simulink model "PMSM_DTC_improved"  (R2022b)
settings: Solver=ode3  StartTime=0.0  StopTime=0.6  FixedStep=5e-6  MaxStep=1e-3  RelTol=1e-4  EnableMultiTasking=on
InitFcn:
  | clear all;
libraries: spsDCVoltageSourceLib x2, spsGroundLib x2, spsPermanentMagnetSynchronousMachineLib x2, spsThreePhaseVIMeasurementLib x2, spsUniversalBridgeLib x2, simulink x1, spsTriangleGeneratorLib x1, sps_lib x1
settings Model: Creator=Administrator  LastModifiedBy=86135
settings SolverCC: AlgebraicLoopSolver=TrustRegion  SolverResetMethod=Robust
settings DataIOCC: LimitDataPoints=on  SaveFormat=Array  SignalLoggingSaveFormat=ModelDataLogs  ReturnWorkspaceOutputs=off
settings OptimizationCC: ExpressionDepthLimit=2147483647  InitFltsAndDblsToZero=on  LifeSpan=inf
settings DebuggingCC: UnderspecifiedInitializationDetection=Classic  MergeDetectMultiDrivingBlocksExec=none  SolverPrmCheckMsg=warning  FcnCallInpInsideContextMsg=warning  UnconnectedInputMsg=warning  UnconnectedOutputMsg=warning  UnconnectedLineMsg=warning  StateNameClashWarn=warning  SFUnexpectedBacktrackingDiag=warning  SFNoUnconditionalDefaultTransitionDiag=warning  SFExecutionAtInitializationDiag=none  SFMachineParentedDataDiag=warning  ArithmeticOperatorsInVariantConditions=warning
settings HardwareCC: ProdBitPerPointer=32  ProdBitPerSizeT=32  ProdBitPerPtrDiffT=32  ProdLargestAtomicFloat=None  ProdIntDivRoundTo=Undefined  ProdEndianess=Unspecified  ProdWordSize=32  ProdHWDeviceType=32-bit Generic
settings ModelReferenceCC: PropagateSignalLabelsOutOfModel=off
settings SFSimCC: SimUseLocalCustomCode=off  CustomCodeUndefinedFunction=UseInterfaceOnly
settings RTWCC: RTWUseLocalCustomCode=off
settings CodeAppCC: StateflowObjectComments=on
settings GRTTargetCC: TargetLangStandard=C89/C90 (ANSI)  CombineOutputUpdateFcns=off  GRTInterface=on
settings ConfigComp: CovMetricSettings=dw  CovSaveCumulativeToWorkspaceVar=on  CovSaveSingleToWorkspaceVar=on  CovExternalEMLEnable=off  CovSFcnEnable=off
settings SimscapeCC: SimscapeNormalizeSystem=off

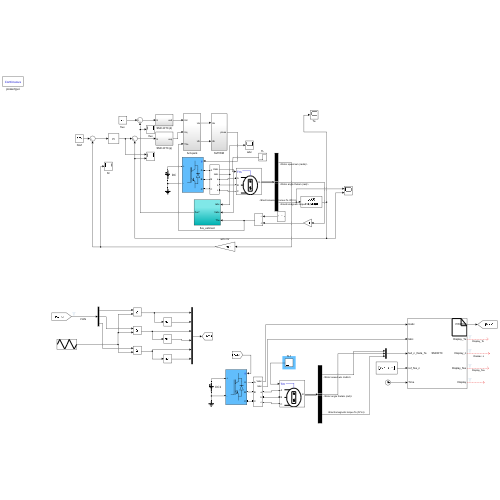
[thumbnail: Simulink's stored preview of the top-level diagram]
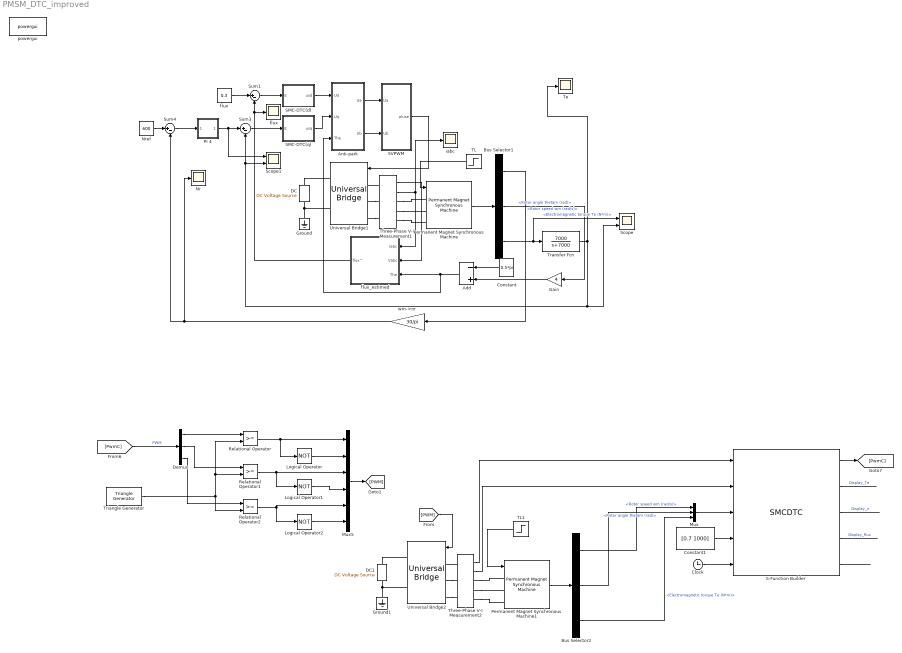
== system PMSM_DTC_improved ==
  Add : Sum  Inputs=-+
  Anti-park : Subsystem
  Bus Selector1 : BusSelector  OutputSignals=Rotor speed wm (rad/s),Rotor angle thetam (rad),Electromagnetic torque Te (N*m)
  Bus Selector2 : BusSelector  OutputSignals=Rotor speed wm (rad/s),Rotor angle thetam (rad),Electromagnetic torque Te (N*m)
  Clock : Clock
  Constant : Constant  Value=0.5*pi
  Constant1 : Constant  Value=[0.7 1000]
  DC : spsDCVoltageSourceLib/DC Voltage Source  Amplitude=311  Measurements=None
  DC1 : spsDCVoltageSourceLib/DC Voltage Source  Amplitude=500  Measurements=None
  Demux : Demux  Outputs=3
  Gain : Gain  Gain=4
  Ground : spsGroundLib/Ground  LConnTagsString=a
  Ground1 : spsGroundLib/Ground  LConnTagsString=a
  Logical Operator : Logic  Operator=NOT  AllPortsSameDT=off  OutDataTypeStr=boolean
  Logical Operator1 : Logic  Operator=NOT  AllPortsSameDT=off  OutDataTypeStr=boolean
  Logical Operator2 : Logic  Operator=NOT  AllPortsSameDT=off  OutDataTypeStr=boolean
  Mux : Mux  Inputs=3
  Mux5 : Mux  Inputs=6
  Nr : Scope
  Nref : Constant  Value=600
  PI 4 : Subsystem
      mask Display: disp('PI')
  Permanent Magnet Synchronous Machine : spsPermanentMagnetSynchronousMachineLib/Permanent Magnet Synchronous Machine  NbPhases=3  FluxDistribution=Sinusoidal  RotorType=Salient-pole  MechanicalLoad=Torque Tm  PresetModel=No  ShowDetailedParameters=on  MeasurementBus=off  Resistance=1.2  Inductance=8.5e-3  dqInductances=[8.5e-3,8.5e-3]  La=0.000835  MachineConstant=Torque Constant (N.m / A_peak)  Flux=0.175  VoltageCst=126.966  TorqueCst=1.05  Flat=120  Mechanical=[0.0008 0 4]  PolePairs=4  InitialConditions=[0,0, 0,0]  InitialConditions5ph=[0 0 0 0 0 0]  RefAngle=90 degrees behind phase A axis (modified Park)  IterativeDiscreteModel=Trapezoidal non iterative  TsBlock=-1  TsPowergui=0
  Permanent Magnet Synchronous Machine1 : spsPermanentMagnetSynchronousMachineLib/Permanent Magnet Synchronous Machine  NbPhases=3  FluxDistribution=Sinusoidal  RotorType=Salient-pole  MechanicalLoad=Torque Tm  PresetModel=No  ShowDetailedParameters=on  MeasurementBus=off  Resistance=1.2  Inductance=8.5e-3  dqInductances=[8.5e-3,8.5e-3]  La=0.000835  MachineConstant=Torque Constant (N.m / A_peak)  Flux=0.175  VoltageCst=126.966  TorqueCst=1.05  Flat=120  Mechanical=[0.0008 0 4]  PolePairs=4  InitialConditions=[0,0, 0,0]  InitialConditions5ph=[0 0 0 0 0 0]  RefAngle=90 degrees behind phase A axis (modified Park)  IterativeDiscreteModel=Trapezoidal non iterative  TsBlock=-1  TsPowergui=0
  Relational Operator : RelationalOperator  OutDataTypeStr=boolean  RndMeth=Simplest  InputSameDT=off
  Relational Operator1 : RelationalOperator  OutDataTypeStr=boolean  RndMeth=Simplest  InputSameDT=off
  Relational Operator2 : RelationalOperator  OutDataTypeStr=boolean  RndMeth=Simplest  InputSameDT=off
  S-Function Builder : S-Function  FunctionName=SMCDTC  SFunctionModules=SMCDTC_wrapper.c ControlFunction InverterController  SFunctionDeploymentMode=off  EnableBusSupport=off  mask(S-Function Builder){}
      mask help: Simulink:masks:SFunctionBuilder_MD
      mask init:
      | val = [[.9  0.75 0.75 1 1 .9 .9 1]',[1 1 0.75 0.75 .9 .9 1 .9]'];try , sys = get_param(gcb,'SfunBuilderFcnName');if isempty(sys), sys = get_param(gcb,'FunctionName'); end,catch, sys = get_param(gcb,'FunctionName'); end
      settings: CopyFcn=set_param(gcbh,'LinkStatus','none')  OpenFcn=sfunctionwizard(gcbh)
      mask Display:
      | plot(val(:,1),val(:,2))
      | disp(sys)
      | port_label('input',1,'Uabc')
      | port_label('input',2,'Iabc')
      | port_label('input',3,'fed_n_theta_Te')
      | port_label('input',4,'ref_flux_n')
      | port_label('input',5,'Time')
      | port_label('output',1,'PWMRef')
      | port_label('output',2,'Display_Te')
      | port_label('output',3,'Display_n')
      | port_label('output',4,'Display_flux')
      | port_label('output',5,'Display')
  SMC-DTC(d) : Subsystem
  SMC-DTC(q) : Subsystem
  SVPWM : Subsystem
  Scope : Scope  NumInputPorts=2
  Scope1 : Scope  NumInputPorts=2
  Sum1 : Sum  Inputs=|+-
  Sum3 : Sum  Inputs=|+-
  Sum4 : Sum  Inputs=|+-
  TL : Step  Time=0.2  After=1.5  SampleTime=0
  TL1 : Step  Time=0.2  After=1.3  SampleTime=0
  Te : Scope
  Three-Phase V-I Measurement1 : spsThreePhaseVIMeasurementLib/Three-Phase V-I Measurement  VoltageMeasurement=phase-to-ground  SetLabelV=off  LabelV=Vabc  Vpu=off  VpuLL=off  CurrentMeasurement=yes  SetLabelI=off  LabelI=Iabc  Ipu=off  Pbase=100e6  Vbase=500e3  OutputType=Complex  PhasorSimulation=off  PSBequivalent=0
  Three-Phase V-I Measurement2 : spsThreePhaseVIMeasurementLib/Three-Phase V-I Measurement  VoltageMeasurement=phase-to-ground  SetLabelV=off  LabelV=Vabc  Vpu=off  VpuLL=off  CurrentMeasurement=yes  SetLabelI=off  LabelI=Iabc  Ipu=off  Pbase=100e6  Vbase=500e3  OutputType=Complex  PhasorSimulation=off  PSBequivalent=0
  Transfer Fcn : TransferFcn  Numerator=[7000]  Denominator=[1 7000]
  Triangle Generator : spsTriangleGeneratorLib/Triangle Generator  Freq=5e3  Phase=90  Ts=0
  Universal Bridge1 : spsUniversalBridgeLib/Universal Bridge  Arms=3  SnubberResistance=1e5  SnubberCapacitance=inf  Device=IGBT / Diodes  Ron=1e-3  Lon=0  ForwardVoltages="[  0  0  ]"  ForwardVoltage=0  GTOparameters=[ 10e-6 , 20e-6 ]  IGBTparameters=[ 1e-6 , 2e-6 ]  Measurements=None  Measurements_2=None  converterType=Rectifier
  Universal Bridge2 : spsUniversalBridgeLib/Universal Bridge  Arms=3  SnubberResistance=1e5  SnubberCapacitance=inf  Device=IGBT / Diodes  Ron=1e-3  Lon=0  ForwardVoltages="[  0  0  ]"  ForwardVoltage=0  GTOparameters=[ 10e-6 , 20e-6 ]  IGBTparameters=[ 1e-6 , 2e-6 ]  Measurements=None  Measurements_2=None  converterType=Rectifier
  flux : Scope
  "flux " : Constant  Value=0.3
  flux_estimed : Subsystem
  iabc : Scope
  powergui : sps_lib/powergui  SimulationMode=Continuous  SampleTime=50e-6  frequency=60  Iterations=50  frequencyindice=0  Pbase=100e6  ErrMax=1e-4  UnitsV=kV  UnitsW=MW  buscounter=0  FunctionMessages=off  echomessages=off  EnableUseOfTLC=off  CurrentSourceSwitches=off  DisableSnubberDevices=off  DisableRonSwitches=off  DisableVfSwitches=off  DisplayEquations=off  AutomaticDiscreteSolvers=off  SolverType=Tustin/Backward Euler (TBE)  Interpol=off  ExternalGateDelay=off  methode=off  Ts=0  x0status=blocks  SPID=off  SwTol=0  HookPort=off  NonlinearTolerance=1e-4  nMaxIteration=100  ContinueOnMaxIteration=off  RestoreLinks=warning  ResistiveCurrentMeasurement=off  Frange=[0:2:500]  Ylog=off  Xlog=on  ShowGrid=off  save=off  variable=ZData  structure=0  ZoomFFT=on  StartTime=0.0  cycles=1  DisplayStyle=1  fundamental=60  FreqAxis=off  MaxFrequency=1000  frequencyindicesteady=1  RmsSteady=1  display=off
  wm->nr : Gain  Gain=30/pi
  wires:
  Anti-park/1(Ua) -> SVPWM/1(Ua)
  Anti-park/2(Ub) -> SVPWM/2(Ub)
  SMC-DTC(d)/1(usd) -> Anti-park/1(Ud)
  "flux "/1 -> Sum1/1
  Sum1/1 -> SMC-DTC(d)/1(E)
  SMC-DTC(q)/1(usq) -> Anti-park/2(Uq)
  Nref/1 -> Sum4/1
  Sum4/1 -> PI 4/1(In1)
  Sum3/1 -> SMC-DTC(q)/1(E)
  wm->nr/1 -> Sum4/2, Nr/1
  TL/1 -> Permanent Magnet Synchronous Machine/1
  SVPWM/1(pluse) -> Universal Bridge1/1
  flux_estimed/1(flux^) -> Sum1/2, flux/1
  Three-Phase V-I Measurement1/1 -> flux_estimed/2(Vabc)
  Gain/1 -> Add/2
  Constant/1 -> Add/1
  Add/1 -> Anti-park/3(The), flux_estimed/3(The)
  Three-Phase V-I Measurement1/2 -> flux_estimed/1(Iabc), iabc/1
  Bus Selector1/3 -> Scope/1, Transfer Fcn/1  "<Electromagnetic torque Te (N*m)>"
  Bus Selector1/2 -> Gain/1  "<Rotor angle thetam (rad)>"
  Bus Selector1/1 -> wm->nr/1  "<Rotor speed wm (rad/s)>"
  Permanent Magnet Synchronous Machine/1 -> Bus Selector1/1
  Permanent Magnet Synchronous Machine1/1 -> Bus Selector2/1
  Three-Phase V-I Measurement2/2 -> S-Function Builder/2
  Bus Selector2/3 -> Mux/3  "<Electromagnetic torque Te (N*m)>"
  TL1/1 -> Permanent Magnet Synchronous Machine1/1
  Bus Selector2/1 -> Mux/1  "<Rotor speed wm (rad/s)>"
  Three-Phase V-I Measurement2/1 -> S-Function Builder/1
  Demux/1 -> Relational Operator/1
  Mux5/1 -> [PWM]
  Relational Operator1/1 -> Mux5/3, Logical Operator1/1
  Logical Operator/1 -> Mux5/2
  Demux/3 -> Relational Operator2/1
  Triangle Generator/1 -> Relational Operator/2, Relational Operator1/2, Relational Operator2/2
  Demux/2 -> Relational Operator1/1
  Relational Operator2/1 -> Mux5/5, Logical Operator2/1
  Logical Operator1/1 -> Mux5/4
  Logical Operator2/1 -> Mux5/6
  Relational Operator/1 -> Mux5/1, Logical Operator/1
  [PwmC] -> Demux/1  "PWM"
  S-Function Builder/1 -> [PwmC]
  Mux/1 -> S-Function Builder/3
  Bus Selector2/2 -> Mux/2  "<Rotor angle thetam (rad)>"
  Constant1/1 -> S-Function Builder/4
  [PWM] -> Universal Bridge2/1
  Clock/1 -> S-Function Builder/5
  S-Function Builder/2 -> ?  "Display_Te"
  S-Function Builder/3 -> ?  "Display_n"
  S-Function Builder/4 -> ?  "Display_flux"
  S-Function Builder/5 -> ?
  Transfer Fcn/1 -> Te/1, Scope1/2, Sum3/2, Scope/2
  PI 4/1(Out1) -> Scope1/1, Sum3/1
  connections:
  Ground/LConn1 -- Universal Bridge1/RConn2 -- DC/LConn1
  Three-Phase V-I Measurement1/RConn1 -- Permanent Magnet Synchronous Machine/LConn1
  DC/RConn1 -- Universal Bridge1/RConn1
  Universal Bridge1/LConn2 -- Three-Phase V-I Measurement1/LConn2
  Three-Phase V-I Measurement1/LConn1 -- Universal Bridge1/LConn1
  Universal Bridge1/LConn3 -- Three-Phase V-I Measurement1/LConn3
  Three-Phase V-I Measurement1/RConn3 -- Permanent Magnet Synchronous Machine/LConn3
  Three-Phase V-I Measurement1/RConn2 -- Permanent Magnet Synchronous Machine/LConn2
  DC1/LConn1 -- Ground1/LConn1 -- Universal Bridge2/RConn2
  Three-Phase V-I Measurement2/LConn1 -- Universal Bridge2/LConn1
  Three-Phase V-I Measurement2/RConn3 -- Permanent Magnet Synchronous Machine1/LConn3
  Universal Bridge2/LConn2 -- Three-Phase V-I Measurement2/LConn2
  Three-Phase V-I Measurement2/RConn1 -- Permanent Magnet Synchronous Machine1/LConn1
  DC1/RConn1 -- Universal Bridge2/RConn1
  Three-Phase V-I Measurement2/RConn2 -- Permanent Magnet Synchronous Machine1/LConn2
  Universal Bridge2/LConn3 -- Three-Phase V-I Measurement2/LConn3

== system PMSM_DTC_improved/Anti-park ==
  Ud : Inport
  Uq : Inport  Port=2
  The : Inport  Port=3
  Fcn : Fcn  Expr=u(1)*cos(u(3))-u(2)*sin(u(3))
  Fcn1 : Fcn  Expr=u(1)*sin(u(3))+u(2)*cos(u(3))
  Mux1 : Mux  Inputs=3
  Ua : Outport
  Ub : Outport  Port=2
  wires:
  Uq/1 -> Mux1/2
  Ud/1 -> Mux1/1
  Fcn1/1 -> Ub/1
  Fcn/1 -> Ua/1
  Mux1/1 -> Fcn1/1, Fcn/1
  The/1 -> Mux1/3

== system PMSM_DTC_improved/PI 4 ==
  In1 : Inport
  Add : Sum
  Gain : Gain  Gain=0.05
  Gain1 : Gain  Gain=20
  Integrator : Integrator
  Saturation : Saturate  UpperLimit=50  LowerLimit=-50
  Out1 : Outport
  wires:
  Gain1/1 -> Integrator/1
  In1/1 -> Gain/1, Gain1/1
  Gain/1 -> Add/1
  Integrator/1 -> Add/2
  Add/1 -> Saturation/1
  Saturation/1 -> Out1/1

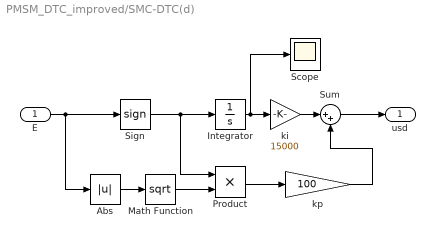
== system PMSM_DTC_improved/SMC-DTC(d) ==
  E : Inport
  Abs : Abs  SaturateOnIntegerOverflow=off
  Integrator : Integrator
  Math Function : Math  Operator=sqrt  SignedPower=on
  Product : Product  RndMeth=Zero
  Scope : Scope
  Sign : Signum
  Sum : Sum  Inputs=|++
  ki : Gain  Gain=15000
  kp : Gain  Gain=100
  usd : Outport
  wires:
  Sum/1 -> usd/1
  E/1 -> Sign/1, Abs/1
  Sign/1 -> Integrator/1, Product/1
  Abs/1 -> Math Function/1
  Math Function/1 -> Product/2
  Product/1 -> kp/1
  kp/1 -> Sum/2
  ki/1 -> Sum/1
  Integrator/1 -> Scope/1, ki/1

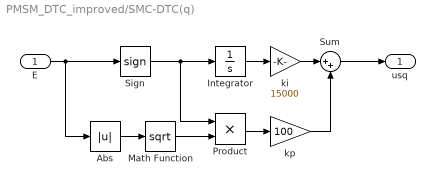
== system PMSM_DTC_improved/SMC-DTC(q) ==
  E : Inport
  Abs : Abs  SaturateOnIntegerOverflow=off
  Integrator : Integrator
  Math Function : Math  Operator=sqrt  SignedPower=on
  Product : Product  RndMeth=Zero
  Sign : Signum
  Sum : Sum  Inputs=|++
  ki : Gain  Gain=15000
  kp : Gain  Gain=100
  usq : Outport
  wires:
  ki/1 -> Sum/1
  kp/1 -> Sum/2
  Product/1 -> kp/1
  Math Function/1 -> Product/2
  Abs/1 -> Math Function/1
  Integrator/1 -> ki/1
  Sign/1 -> Product/1, Integrator/1
  E/1 -> Abs/1, Sign/1
  Sum/1 -> usq/1

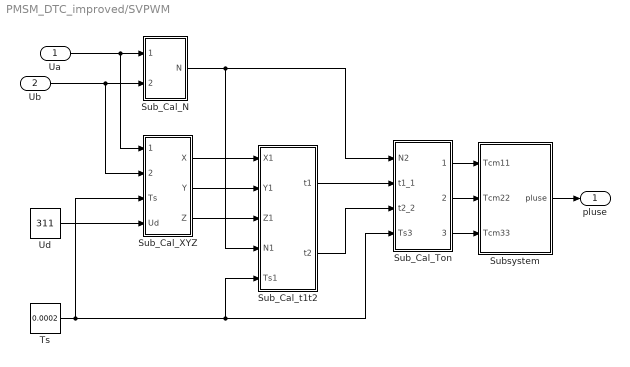
== system PMSM_DTC_improved/SVPWM ==
  Ua : Inport
  Ub : Inport  Port=2
  Sub_Cal_N : Subsystem
  Sub_Cal_Ton : Subsystem
  Sub_Cal_XYZ : Subsystem
  Sub_Cal_t1t2 : Subsystem
  Subsystem : Subsystem
  Ts : Constant  Value=0.0002
  Ud : Constant  Value=311
  pluse : Outport
  wires:
  Ua/1 -> Sub_Cal_N/1(Ualfa), Sub_Cal_XYZ/1(Ualfa1)
  Ub/1 -> Sub_Cal_N/2(Ubeta), Sub_Cal_XYZ/2(Ubeta1)
  Sub_Cal_XYZ/1(X) -> Sub_Cal_t1t2/1(X1)
  Sub_Cal_XYZ/2(Y) -> Sub_Cal_t1t2/2(Y1)
  Sub_Cal_XYZ/3(Z) -> Sub_Cal_t1t2/3(Z1)
  Sub_Cal_t1t2/1(t1) -> Sub_Cal_Ton/2(t1_1)
  Sub_Cal_Ton/1(Tcm1) -> Subsystem/1(Tcm11)
  Sub_Cal_Ton/2(Tcm2) -> Subsystem/2(Tcm22)
  Ts/1 -> Sub_Cal_Ton/4(Ts3), Sub_Cal_t1t2/5(Ts1), Sub_Cal_XYZ/3(Ts)
  Sub_Cal_Ton/3(Tcm3) -> Subsystem/3(Tcm33)
  Subsystem/1(pluse) -> pluse/1
  Sub_Cal_t1t2/2(t2) -> Sub_Cal_Ton/3(t2_2)
  Ud/1 -> Sub_Cal_XYZ/4(Ud)
  Sub_Cal_N/1(N) -> Sub_Cal_Ton/1(N2), Sub_Cal_t1t2/4(N1)

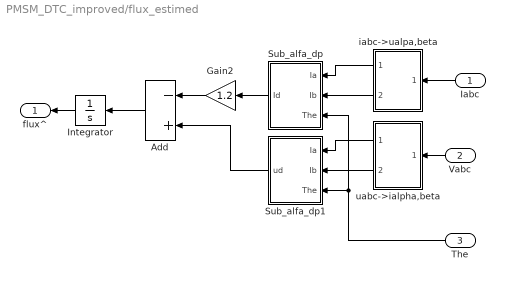
== system PMSM_DTC_improved/flux_estimed ==
  Iabc : Inport
  Vabc : Inport  Port=2
  The : Inport  Port=3
  Add : Sum  Inputs=-+
  Gain2 : Gain  Gain=1.2
  Integrator : Integrator
  Sub_alfa_dp : Subsystem
  Sub_alfa_dp1 : Subsystem
  iabc->ualpa,beta : Subsystem
  uabc->ialpha,beta : Subsystem
  flux^ : Outport
  wires:
  iabc->ualpa,beta/1(ialfa) -> Sub_alfa_dp/1(Ia)
  iabc->ualpa,beta/2(ibeta) -> Sub_alfa_dp/2(Ib)
  uabc->ialpha,beta/1(ualfa) -> Sub_alfa_dp1/1(Ia)
  uabc->ialpha,beta/2(ubeta) -> Sub_alfa_dp1/2(Ib)
  Sub_alfa_dp1/1(ud) -> Add/2
  Sub_alfa_dp/1(Id) -> Gain2/1
  Gain2/1 -> Add/1
  Add/1 -> Integrator/1
  Iabc/1 -> iabc->ualpa,beta/1(iabc)
  Integrator/1 -> flux^/1
  Vabc/1 -> uabc->ialpha,beta/1(uabc)
  The/1 -> Sub_alfa_dp1/3(The), Sub_alfa_dp/3(The)

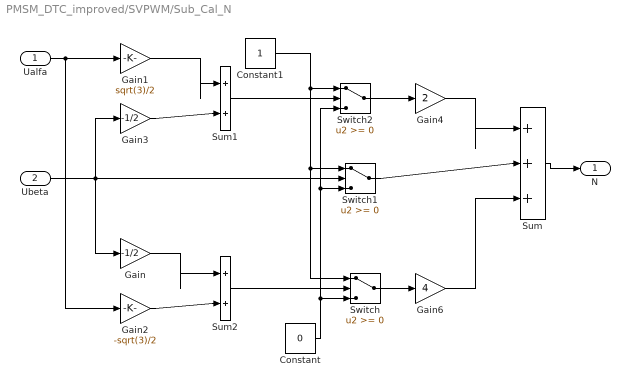
== system PMSM_DTC_improved/SVPWM/Sub_Cal_N ==
  Ualfa : Inport
  Ubeta : Inport  Port=2
  Constant : Constant  Value=0
  Constant1 : Constant
  Gain : Gain  Gain=-1/2
  Gain1 : Gain  Gain=sqrt(3)/2
  Gain2 : Gain  Gain=-sqrt(3)/2
  Gain3 : Gain  Gain=-1/2
  Gain4 : Gain  Gain=2
  Gain6 : Gain  Gain=4
  Sum : Sum  Inputs=|+++
  Sum1 : Sum  Inputs=|++
  Sum2 : Sum  Inputs=|++
  Switch : Switch  SaturateOnIntegerOverflow=off  InputSameDT=off
  Switch1 : Switch  SaturateOnIntegerOverflow=off  InputSameDT=off
  Switch2 : Switch  SaturateOnIntegerOverflow=off  InputSameDT=off
  N : Outport
  wires:
  Ubeta/1 -> Switch1/2, Gain3/1, Gain/1
  Gain1/1 -> Sum1/1
  Gain3/1 -> Sum1/2
  Sum1/1 -> Switch2/2
  Ualfa/1 -> Gain1/1, Gain2/1
  Gain/1 -> Sum2/1
  Gain2/1 -> Sum2/2
  Sum2/1 -> Switch/2
  Constant1/1 -> Switch/1, Switch1/1, Switch2/1
  Constant/1 -> Switch2/3, Switch1/3, Switch/3
  Switch/1 -> Gain6/1
  Switch2/1 -> Gain4/1
  Gain4/1 -> Sum/1
  Switch1/1 -> Sum/2
  Gain6/1 -> Sum/3
  Sum/1 -> N/1

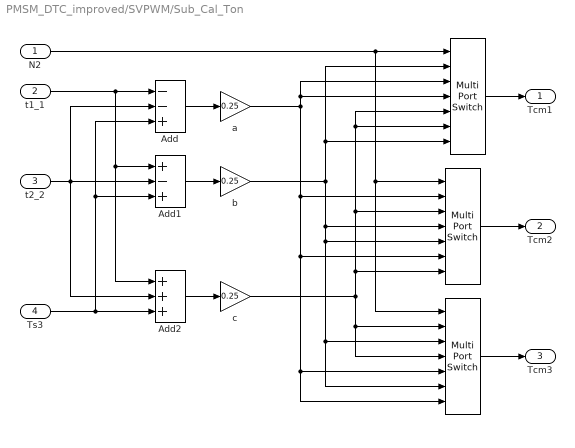
== system PMSM_DTC_improved/SVPWM/Sub_Cal_Ton ==
  N2 : Inport
  t1_1 : Inport  Port=2
  t2_2 : Inport  Port=3
  Ts3 : Inport  Port=4
  " " : MultiPortSwitch  Inputs=6  SaturateOnIntegerOverflow=off  InputSameDT=off
  "  " : MultiPortSwitch  Inputs=6  SaturateOnIntegerOverflow=off  InputSameDT=off
  "    " : MultiPortSwitch  Inputs=6  SaturateOnIntegerOverflow=off  InputSameDT=off
  Add : Sum  Inputs=--+
  Add1 : Sum  Inputs=+-+
  Add2 : Sum  Inputs=+++
  a : Gain  Gain=0.25
  b : Gain  Gain=0.25
  c : Gain  Gain=0.25
  Tcm1 : Outport
  Tcm2 : Outport  Port=2
  Tcm3 : Outport  Port=3
  wires:
  N2/1 -> "  "/1, " "/1, "    "/1
  t1_1/1 -> Add/1, Add1/1, Add2/1
  t2_2/1 -> Add/2, Add1/2, Add2/2
  Ts3/1 -> Add/3, Add1/3, Add2/3
  Add/1 -> a/1
  Add1/1 -> b/1
  Add2/1 -> c/1
  "  "/1 -> Tcm1/1
  " "/1 -> Tcm2/1
  "    "/1 -> Tcm3/1
  b/1 -> "  "/7, "  "/2, " "/4, " "/5, "    "/3, "    "/6
  a/1 -> " "/2, " "/6, "    "/5, "    "/7, "  "/4, "  "/3
  c/1 -> "  "/5, "  "/6, " "/3, " "/7, "    "/2, "    "/4

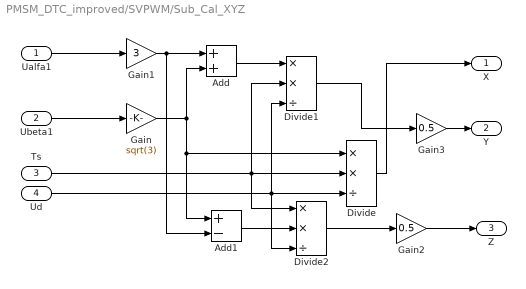
== system PMSM_DTC_improved/SVPWM/Sub_Cal_XYZ ==
  Ualfa1 : Inport
  Ubeta1 : Inport  Port=2
  Ts : Inport  Port=3
  Ud : Inport  Port=4
  Add : Sum
  Add1 : Sum  Inputs=+-
  Divide : Product  Inputs=**/
  Divide1 : Product  Inputs=**/
  Divide2 : Product  Inputs=**/
  Gain : Gain  Gain=sqrt(3)
  Gain1 : Gain  Gain=3
  Gain2 : Gain  Gain=0.5
  Gain3 : Gain  Gain=0.5
  X : Outport
  Y : Outport  Port=2
  Z : Outport  Port=3
  wires:
  Ubeta1/1 -> Gain/1
  Gain/1 -> Add/2, Divide/1, Add1/1
  Ts/1 -> Divide/2, Divide1/2, Divide2/1
  Ud/1 -> Divide/3, Divide1/3, Divide2/3
  Ualfa1/1 -> Gain1/1
  Gain1/1 -> Add/1, Add1/2
  Add/1 -> Divide1/1
  Add1/1 -> Divide2/2
  Divide2/1 -> Gain2/1
  Gain2/1 -> Z/1
  Divide/1 -> X/1
  Divide1/1 -> Gain3/1
  Gain3/1 -> Y/1

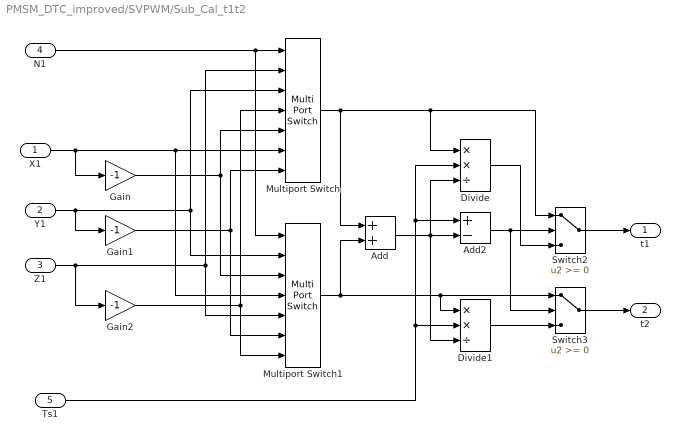
== system PMSM_DTC_improved/SVPWM/Sub_Cal_t1t2 ==
  X1 : Inport
  Y1 : Inport  Port=2
  Z1 : Inport  Port=3
  N1 : Inport  Port=4
  Ts1 : Inport  Port=5
  Add : Sum
  Add2 : Sum  Inputs=+-
  Divide : Product  Inputs=**/
  Divide1 : Product  Inputs=**/
  Gain : Gain  Gain=-1
  Gain1 : Gain  Gain=-1
  Gain2 : Gain  Gain=-1
  Multiport Switch : MultiPortSwitch  Inputs=6  SaturateOnIntegerOverflow=off  InputSameDT=off
  Multiport Switch1 : MultiPortSwitch  Inputs=6  SaturateOnIntegerOverflow=off  InputSameDT=off
  Switch2 : Switch  SaturateOnIntegerOverflow=off  InputSameDT=off
  Switch3 : Switch  SaturateOnIntegerOverflow=off  InputSameDT=off
  t1 : Outport
  t2 : Outport  Port=2
  wires:
  N1/1 -> Multiport Switch/1, Multiport Switch1/1
  Y1/1 -> Gain1/1, Multiport Switch/3, Multiport Switch1/2
  X1/1 -> Gain/1, Multiport Switch/6, Multiport Switch1/4
  Z1/1 -> Gain2/1, Multiport Switch/2, Multiport Switch1/5
  Multiport Switch/1 -> Add/1, Divide/1, Switch2/1
  Multiport Switch1/1 -> Add/2, Switch3/1, Divide1/1
  Ts1/1 -> Divide1/2, Divide/2, Add2/1
  Add2/1 -> Switch2/2, Switch3/2
  Divide/1 -> Switch2/3
  Divide1/1 -> Switch3/3
  Switch3/1 -> t2/1
  Switch2/1 -> t1/1
  Add/1 -> Divide/3, Divide1/3, Add2/2
  Gain1/1 -> Multiport Switch1/6, Multiport Switch/7
  Gain2/1 -> Multiport Switch/4, Multiport Switch1/7
  Gain/1 -> Multiport Switch/5, Multiport Switch1/3

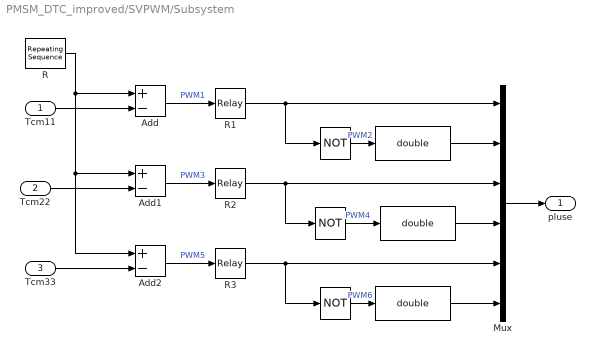
== system PMSM_DTC_improved/SVPWM/Subsystem ==
  Tcm11 : Inport
  Tcm22 : Inport  Port=2
  Tcm33 : Inport  Port=3
  " " : Logic  Operator=NOT  AllPortsSameDT=off  OutDataTypeStr=boolean
  "  " : DataTypeConversion  OutDataTypeStr=double  SaturateOnIntegerOverflow=off  RndMeth=Floor
  "   " : Logic  Operator=NOT  AllPortsSameDT=off  OutDataTypeStr=boolean
  "     " : DataTypeConversion  OutDataTypeStr=double  SaturateOnIntegerOverflow=off  RndMeth=Floor
  "       " : Logic  Operator=NOT  AllPortsSameDT=off  OutDataTypeStr=boolean
  "         " : DataTypeConversion  OutDataTypeStr=double  SaturateOnIntegerOverflow=off  RndMeth=Floor
  Add : Sum  Inputs=+-
  Add1 : Sum  Inputs=+-
  Add2 : Sum  Inputs=+-
  Mux : Mux  Inputs=6
  R : simulink/Sources/Repeating Sequence  rep_seq_t="[0  0.0001  0.0002]"  rep_seq_y="[0  0.0001  0]"
  R1 : Relay
  R2 : Relay
  R3 : Relay
  pluse : Outport
  wires:
  "  "/1 -> Mux/2
  "     "/1 -> Mux/4
  "         "/1 -> Mux/6
  R2/1 -> Mux/3, "   "/1
  R3/1 -> Mux/5, "       "/1
  R1/1 -> Mux/1, " "/1
  Mux/1 -> pluse/1
  "       "/1 -> "         "/1  "PWM6"
  "   "/1 -> "     "/1  "PWM4"
  " "/1 -> "  "/1  "PWM2"
  Add2/1 -> R3/1  "PWM5"
  Add1/1 -> R2/1  "PWM3"
  Add/1 -> R1/1  "PWM1"
  R/1 -> Add/1, Add1/1, Add2/1
  Tcm33/1 -> Add2/2
  Tcm22/1 -> Add1/2
  Tcm11/1 -> Add/2

== system PMSM_DTC_improved/flux_estimed/Sub_alfa_dp ==
  Ia : Inport
  Ib : Inport  Port=2
  The : Inport  Port=3
  Fcn : Fcn  Expr=cos(u)
  Fcn1 : Fcn  Expr=sin(u)
  Fcn2 : Fcn  Expr=u(1)*u(3)+u(2)*u(4)
  Mux : Mux
  Id : Outport
  wires:
  The/1 -> Fcn/1, Fcn1/1
  Ia/1 -> Mux/1
  Ib/1 -> Mux/2
  Fcn/1 -> Mux/3
  Fcn1/1 -> Mux/4
  Mux/1 -> Fcn2/1
  Fcn2/1 -> Id/1

== system PMSM_DTC_improved/flux_estimed/Sub_alfa_dp1 ==
  Ia : Inport
  Ib : Inport  Port=2
  The : Inport  Port=3
  Fcn : Fcn  Expr=cos(u)
  Fcn1 : Fcn  Expr=sin(u)
  Fcn2 : Fcn  Expr=u(1)*u(3)+u(2)*u(4)
  Mux : Mux
  ud : Outport
  wires:
  Fcn2/1 -> ud/1
  Mux/1 -> Fcn2/1
  Fcn1/1 -> Mux/4
  Fcn/1 -> Mux/3
  Ib/1 -> Mux/2
  Ia/1 -> Mux/1
  The/1 -> Fcn1/1, Fcn/1

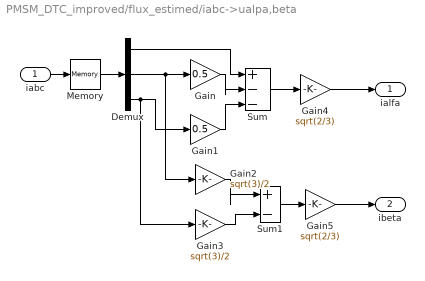
== system PMSM_DTC_improved/flux_estimed/iabc->ualpa,beta ==
  iabc : Inport
  Demux : Demux  Outputs=3
  Gain : Gain  Gain=0.5
  Gain1 : Gain  Gain=0.5
  Gain2 : Gain  Gain=sqrt(3)/2
  Gain3 : Gain  Gain=sqrt(3)/2
  Gain4 : Gain  Gain=sqrt(2/3)
  Gain5 : Gain  Gain=sqrt(2/3)
  Memory : Memory
  Sum : Sum  Inputs=|+--
  Sum1 : Sum  Inputs=|+-
  ialfa : Outport
  ibeta : Outport  Port=2
  wires:
  iabc/1 -> Memory/1
  Demux/2 -> Gain/1, Gain2/1
  Sum/1 -> Gain4/1
  Sum1/1 -> Gain5/1
  Demux/1 -> Sum/1
  Demux/3 -> Gain1/1, Gain3/1
  Gain2/1 -> Sum1/1
  Gain3/1 -> Sum1/2
  Gain/1 -> Sum/2
  Gain1/1 -> Sum/3
  Gain4/1 -> ialfa/1
  Gain5/1 -> ibeta/1
  Memory/1 -> Demux/1

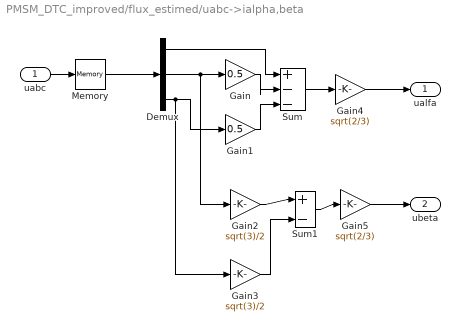
== system PMSM_DTC_improved/flux_estimed/uabc->ialpha,beta ==
  uabc : Inport
  Demux : Demux  Outputs=3
  Gain : Gain  Gain=0.5
  Gain1 : Gain  Gain=0.5
  Gain2 : Gain  Gain=sqrt(3)/2
  Gain3 : Gain  Gain=sqrt(3)/2
  Gain4 : Gain  Gain=sqrt(2/3)
  Gain5 : Gain  Gain=sqrt(2/3)
  Memory : Memory
  Sum : Sum  Inputs=|+--
  Sum1 : Sum  Inputs=|+-
  ualfa : Outport
  ubeta : Outport  Port=2
  wires:
  uabc/1 -> Memory/1
  Demux/2 -> Gain/1, Gain2/1
  Sum/1 -> Gain4/1
  Sum1/1 -> Gain5/1
  Demux/1 -> Sum/1
  Demux/3 -> Gain1/1, Gain3/1
  Gain2/1 -> Sum1/1
  Gain3/1 -> Sum1/2
  Gain/1 -> Sum/2
  Gain1/1 -> Sum/3
  Gain4/1 -> ualfa/1
  Gain5/1 -> ubeta/1
  Memory/1 -> Demux/1
